simulink model "Actuators"  (Simulink 8.4)
settings: Solver=ode45  StartTime=0.0  StopTime=10.0  RelTol=1e-3
undefined symbols (not defined in the file): Ais_flgAirInjReacPumpOverride, Ais_stAirInjReacPumpMan, Apv_facAirPumpRateMan, Apv_factor, Apv_flgAirPumpRateOverride, Apv_tiPeriod_C, CDRV_E_OK_, Cov_facChOverVlvRateMan, Cov_factor, Cov_flgChOverVlvRateOverride, Cov_tiPeriod_C, Doh_OutputDiagnosisOverride, Fps_flgFuelPumpOverride, Fps_stFuelPumpMan, Icc_degIgnMan, Icc_flgIgnAngleOverride, Icc_flgIgnCutoffMan, Icc_flgIgnCutoffOverride, Icc_nrFollowUpSparks, Icc_tiDwell, Icc_tiDwellFollowUpSparks, Icc_tiOffFollowUpSparks, Ics_flgIntercoolerOverride, Ics_stIntercoolerMan, Ivc_degInjAbort, Ivc_degIntakeClose, Ivc_degOffsetInjEndSimultanInj, Ivc_flgBattDelayOverride, Ivc_flgDiagEntryCondFulfilled, Ivc_flgEndOfStartCond, Ivc_flgInjCutoff, Ivc_flgInjCutoffOverride, Ivc_flgInjTimeOverride, Ivc_flgOverrunCutoff, Ivc_flgPostInjCond, Ivc_tiBattDelayMan, Ivc_tiInjEff, Ivc_tiInjMan, Ivc_tiMinThresDeltaEffInjPeriod, Ivc_weea0, Ivc_weea1, Ivc_weea2, Lo_, Mrs_flgMainRelaisOverride, Mrs_stMainRelaisMan, Normal, OK, OpenCircuit, OverTemp, ShortToBatt, ShortToBattNEG, ShortToGnd, ShortToGndNEG, ShortToGndPOS, Str_flgStarterOverride, Str_stStarterMan, Tvc_facDutycyclePIDLimitMax, Tvc_facDutycyclePIDLimitMin, Tvc_facDutycyclePilotControlNeg, Tvc_facDutycyclePilotControlPos ... (+20)
libraries: simulink x9
(part 2 of 3)

== system Actuators/Actuators_mdl/Apv/G1_PWM_Output_Ctrl ==
  dutycycle : Inport
  period : Inport  Port=2
  factor : Inport  Port=3
  level : Inport  Port=4
  DTC_PwmOut_DutyCycle : DataTypeConversion  OutDataTypeStr=int16  RndMeth=Nearest
  DTC_PwmOut_ErrorInfo : DataTypeConversion  OutDataTypeStr=boolean
  DTC_PwmOut_Level : DataTypeConversion  OutDataTypeStr=int16  RndMeth=Nearest
  DTC_PwmOut_Period : DataTypeConversion  OutDataTypeStr=int16  RndMeth=Nearest
  DTC_PwmOut_Period1 : DataTypeConversion  OutDataTypeStr=uint8  RndMeth=Nearest
  FlexECU_DevLib_FcnAPI_Wrapper_SFcn : S-Function  FunctionName=ehooks_medc17flex_devlib_basic_io_fcncall  Parameters=NoInputPorts, NoOutputPorts, InputPortDataTypes, OutputPortDataTypes, CFunctionArgTypes, CFunctionName, ChannelName  EnableBusSupport=off  mask{NoInputPorts=4, NoOutputPorts=1, InputPortDataTypes=int16,int16, int16, uint8, OutputPortDataTypes=uint8, CFunctionArgTypes=ret,val,val,val,val, CFunctionName=DevLib_Pwm_Out, ChannelName=O_T_RL13}
      mask prompts: NoInputPorts "Number of input ports"; NoOutputPorts "Number of output ports"; InputPortDataTypes "Input port data types"; OutputPortDataTypes "Output port data types"; CFunctionArgTypes "C function argument types"; CFunctionName "C function name"; ChannelName "Channel (pin) name"
      mask Display: disp('EHOOKS FlexECU\nDevLib Wrapper\nS-Function')
  Gain : Gain  Gain=100
  status : Outport
  wires:
  DTC_PwmOut_ErrorInfo/1 -> status/1
  DTC_PwmOut_Level/1 -> FlexECU_DevLib_FcnAPI_Wrapper_SFcn/3
  DTC_PwmOut_Period/1 -> FlexECU_DevLib_FcnAPI_Wrapper_SFcn/2
  DTC_PwmOut_DutyCycle/1 -> FlexECU_DevLib_FcnAPI_Wrapper_SFcn/1
  factor/1 -> DTC_PwmOut_Level/1
  period/1 -> DTC_PwmOut_Period/1
  FlexECU_DevLib_FcnAPI_Wrapper_SFcn/1 -> DTC_PwmOut_ErrorInfo/1
  DTC_PwmOut_Period1/1 -> FlexECU_DevLib_FcnAPI_Wrapper_SFcn/4
  level/1 -> DTC_PwmOut_Period1/1
  dutycycle/1 -> Gain/1
  Gain/1 -> DTC_PwmOut_DutyCycle/1

== system Actuators/Actuators_mdl/Apv/G1_PwmOut_Get_error ==
  DTC_PwmOut_GetError : DataTypeConversion  OutDataTypeStr=single
  FlexECU_DevLib_FcnAPI_Wrapper_SFcn : S-Function  FunctionName=ehooks_medc17flex_devlib_basic_io_fcncall  Parameters=NoInputPorts, NoOutputPorts, InputPortDataTypes, OutputPortDataTypes, CFunctionArgTypes, CFunctionName, ChannelName  EnableBusSupport=off  mask{NoInputPorts=0, NoOutputPorts=1, InputPortDataTypes=, OutputPortDataTypes=uint8, CFunctionArgTypes=ret, CFunctionName=DevLib_PwmOut_GetError, ChannelName=O_T_RL13}
      mask prompts: NoInputPorts "Number of input ports"; NoOutputPorts "Number of output ports"; InputPortDataTypes "Input port data types"; OutputPortDataTypes "Output port data types"; CFunctionArgTypes "C function argument types"; CFunctionName "C function name"; ChannelName "Channel (pin) name"
      mask Display: disp('EHOOKS FlexECU\nDevLib Wrapper\nS-Function')
  status : Outport
  wires:
  FlexECU_DevLib_FcnAPI_Wrapper_SFcn/1 -> DTC_PwmOut_GetError/1
  DTC_PwmOut_GetError/1 -> status/1

== system Actuators/Actuators_mdl/Cov/G1_PWM_Output_Ctrl ==
  dutycycle : Inport
  period : Inport  Port=2
  factor : Inport  Port=3
  level : Inport  Port=4
  DTC_PwmOut_DutyCycle : DataTypeConversion  OutDataTypeStr=int16  RndMeth=Nearest
  DTC_PwmOut_ErrorInfo : DataTypeConversion  OutDataTypeStr=boolean
  DTC_PwmOut_Level : DataTypeConversion  OutDataTypeStr=int16  RndMeth=Nearest
  DTC_PwmOut_Period : DataTypeConversion  OutDataTypeStr=int16  RndMeth=Nearest
  DTC_PwmOut_Period1 : DataTypeConversion  OutDataTypeStr=uint8  RndMeth=Nearest
  FlexECU_DevLib_FcnAPI_Wrapper_SFcn : S-Function  FunctionName=ehooks_medc17flex_devlib_basic_io_fcncall  Parameters=NoInputPorts, NoOutputPorts, InputPortDataTypes, OutputPortDataTypes, CFunctionArgTypes, CFunctionName, ChannelName  EnableBusSupport=off  mask{NoInputPorts=4, NoOutputPorts=1, InputPortDataTypes=int16,int16, int16, uint8, OutputPortDataTypes=uint8, CFunctionArgTypes=ret,val,val,val,val, CFunctionName=DevLib_Pwm_Out, ChannelName=O_T_RL10}
      mask prompts: NoInputPorts "Number of input ports"; NoOutputPorts "Number of output ports"; InputPortDataTypes "Input port data types"; OutputPortDataTypes "Output port data types"; CFunctionArgTypes "C function argument types"; CFunctionName "C function name"; ChannelName "Channel (pin) name"
      mask Display: disp('EHOOKS FlexECU\nDevLib Wrapper\nS-Function')
  Gain : Gain  Gain=100
  status : Outport
  wires:
  Gain/1 -> DTC_PwmOut_DutyCycle/1
  dutycycle/1 -> Gain/1
  level/1 -> DTC_PwmOut_Period1/1
  DTC_PwmOut_Period1/1 -> FlexECU_DevLib_FcnAPI_Wrapper_SFcn/4
  FlexECU_DevLib_FcnAPI_Wrapper_SFcn/1 -> DTC_PwmOut_ErrorInfo/1
  period/1 -> DTC_PwmOut_Period/1
  factor/1 -> DTC_PwmOut_Level/1
  DTC_PwmOut_DutyCycle/1 -> FlexECU_DevLib_FcnAPI_Wrapper_SFcn/1
  DTC_PwmOut_Period/1 -> FlexECU_DevLib_FcnAPI_Wrapper_SFcn/2
  DTC_PwmOut_Level/1 -> FlexECU_DevLib_FcnAPI_Wrapper_SFcn/3
  DTC_PwmOut_ErrorInfo/1 -> status/1

== system Actuators/Actuators_mdl/Cov/G1_PwmOut_Get_error ==
  DTC_PwmOut_GetError : DataTypeConversion  OutDataTypeStr=single
  FlexECU_DevLib_FcnAPI_Wrapper_SFcn : S-Function  FunctionName=ehooks_medc17flex_devlib_basic_io_fcncall  Parameters=NoInputPorts, NoOutputPorts, InputPortDataTypes, OutputPortDataTypes, CFunctionArgTypes, CFunctionName, ChannelName  EnableBusSupport=off  mask{NoInputPorts=0, NoOutputPorts=1, InputPortDataTypes=, OutputPortDataTypes=uint8, CFunctionArgTypes=ret, CFunctionName=DevLib_PwmOut_GetError, ChannelName=O_T_RL10}
      mask prompts: NoInputPorts "Number of input ports"; NoOutputPorts "Number of output ports"; InputPortDataTypes "Input port data types"; OutputPortDataTypes "Output port data types"; CFunctionArgTypes "C function argument types"; CFunctionName "C function name"; ChannelName "Channel (pin) name"
      mask Display: disp('EHOOKS FlexECU\nDevLib Wrapper\nS-Function')
  status : Outport
  wires:
  DTC_PwmOut_GetError/1 -> status/1
  FlexECU_DevLib_FcnAPI_Wrapper_SFcn/1 -> DTC_PwmOut_GetError/1

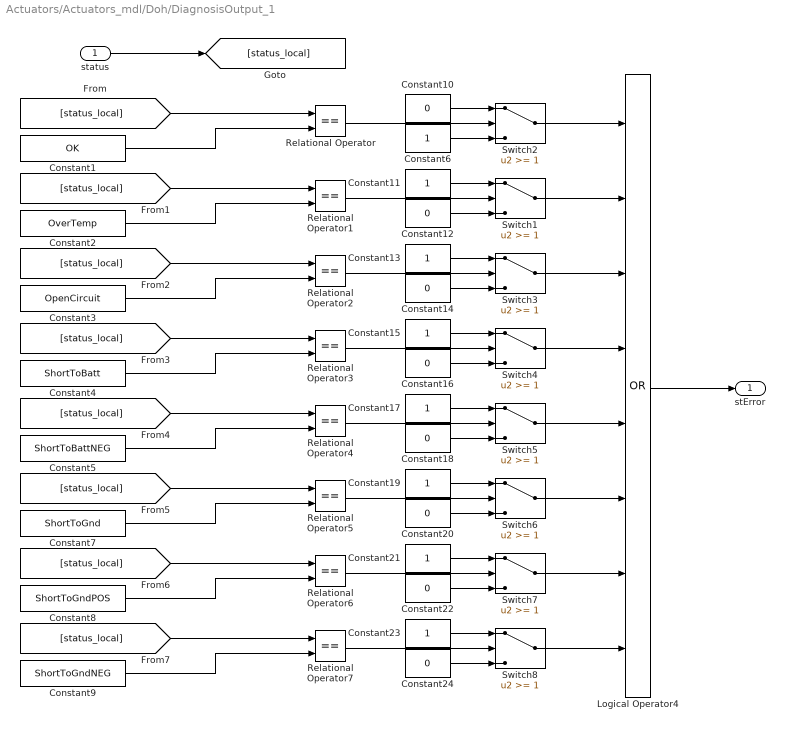
== system Actuators/Actuators_mdl/Doh/DiagnosisOutput_1 ==
  status : Inport
  Constant1 : Constant  Value=OK
  Constant{10,12,14,16,18,20,22,24} (8 alike) : Constant  Value=0  OutDataTypeStr=boolean
  Constant{6,11,13,15,17,19,21,23} (8 alike) : Constant  OutDataTypeStr=boolean
  Constant2 : Constant  Value=OverTemp
  Constant3 : Constant  Value=OpenCircuit
  Constant4 : Constant  Value=ShortToBatt
  Constant5 : Constant  Value=ShortToBattNEG
  Constant7 : Constant  Value=ShortToGnd
  Constant8 : Constant  Value=ShortToGndPOS
  Constant9 : Constant  Value=ShortToGndNEG
  Logical Operator4 : Logic  Operator=OR  Inputs=8  AllPortsSameDT=off  OutDataTypeStr=boolean
  Relational Operator{,1..7} (8 alike) : RelationalOperator  Operator===  OutDataTypeStr=boolean
  Switch{1..8} (8 alike) : Switch  Threshold=1
  stError : Outport
  wires:
  Constant1/1 -> Relational Operator/2
  status/1 -> [status_local]
  [status_local] -> Relational Operator/1
  Constant2/1 -> Relational Operator1/2
  [status_local] -> Relational Operator1/1
  Constant3/1 -> Relational Operator2/2
  [status_local] -> Relational Operator2/1
  Constant4/1 -> Relational Operator3/2
  [status_local] -> Relational Operator3/1
  Constant5/1 -> Relational Operator4/2
  [status_local] -> Relational Operator4/1
  Constant7/1 -> Relational Operator5/2
  [status_local] -> Relational Operator5/1
  Constant8/1 -> Relational Operator6/2
  [status_local] -> Relational Operator6/1
  Constant9/1 -> Relational Operator7/2
  [status_local] -> Relational Operator7/1
  Relational Operator/1 -> Switch2/2
  Constant6/1 -> Switch2/3
  Logical Operator4/1 -> stError/1
  Constant10/1 -> Switch2/1
  Constant12/1 -> Switch1/3
  Constant11/1 -> Switch1/1
  Relational Operator1/1 -> Switch1/2
  Constant14/1 -> Switch3/3
  Constant13/1 -> Switch3/1
  Relational Operator2/1 -> Switch3/2
  Constant16/1 -> Switch4/3
  Constant15/1 -> Switch4/1
  Relational Operator3/1 -> Switch4/2
  Constant18/1 -> Switch5/3
  Constant17/1 -> Switch5/1
  Relational Operator4/1 -> Switch5/2
  Constant20/1 -> Switch6/3
  Constant19/1 -> Switch6/1
  Relational Operator5/1 -> Switch6/2
  Constant22/1 -> Switch7/3
  Constant21/1 -> Switch7/1
  Relational Operator6/1 -> Switch7/2
  Constant24/1 -> Switch8/3
  Constant23/1 -> Switch8/1
  Relational Operator7/1 -> Switch8/2
  Switch2/1 -> Logical Operator4/1
  Switch1/1 -> Logical Operator4/2
  Switch3/1 -> Logical Operator4/3
  Switch4/1 -> Logical Operator4/4
  Switch5/1 -> Logical Operator4/5
  Switch6/1 -> Logical Operator4/6
  Switch7/1 -> Logical Operator4/7
  Switch8/1 -> Logical Operator4/8

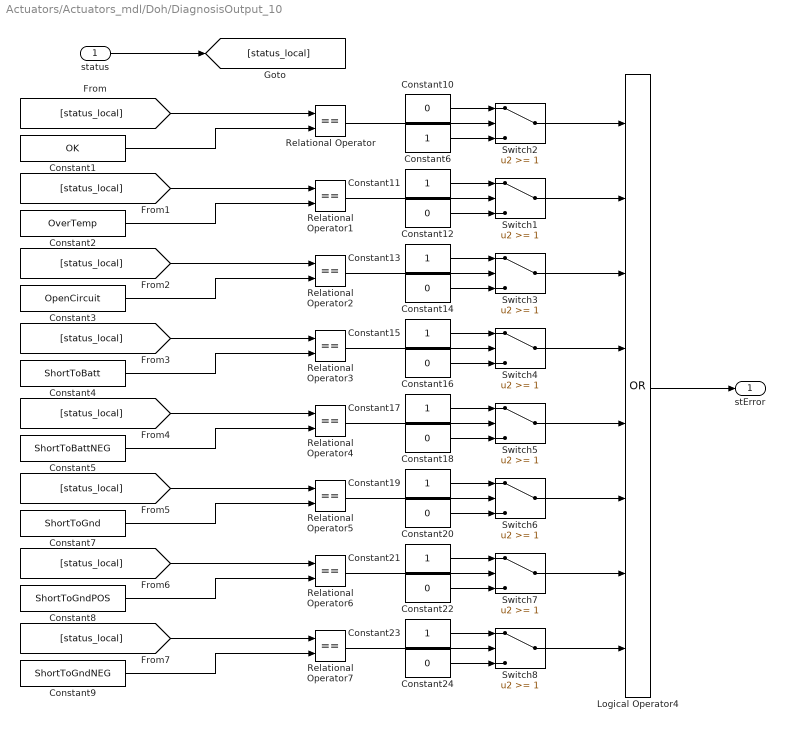
== system Actuators/Actuators_mdl/Doh/DiagnosisOutput_10 ==
  status : Inport
  Constant1 : Constant  Value=OK
  Constant{10,12,14,16,18,20,22,24} (8 alike) : Constant  Value=0  OutDataTypeStr=boolean
  Constant{6,11,13,15,17,19,21,23} (8 alike) : Constant  OutDataTypeStr=boolean
  Constant2 : Constant  Value=OverTemp
  Constant3 : Constant  Value=OpenCircuit
  Constant4 : Constant  Value=ShortToBatt
  Constant5 : Constant  Value=ShortToBattNEG
  Constant7 : Constant  Value=ShortToGnd
  Constant8 : Constant  Value=ShortToGndPOS
  Constant9 : Constant  Value=ShortToGndNEG
  Logical Operator4 : Logic  Operator=OR  Inputs=8  AllPortsSameDT=off  OutDataTypeStr=boolean
  Relational Operator{,1..7} (8 alike) : RelationalOperator  Operator===  OutDataTypeStr=boolean
  Switch{1..8} (8 alike) : Switch  Threshold=1
  stError : Outport
  wires:
  Switch8/1 -> Logical Operator4/8
  Switch7/1 -> Logical Operator4/7
  Switch6/1 -> Logical Operator4/6
  Switch5/1 -> Logical Operator4/5
  Switch4/1 -> Logical Operator4/4
  Switch3/1 -> Logical Operator4/3
  Switch1/1 -> Logical Operator4/2
  Switch2/1 -> Logical Operator4/1
  Relational Operator7/1 -> Switch8/2
  Constant23/1 -> Switch8/1
  Constant24/1 -> Switch8/3
  Relational Operator6/1 -> Switch7/2
  Constant21/1 -> Switch7/1
  Constant22/1 -> Switch7/3
  Relational Operator5/1 -> Switch6/2
  Constant19/1 -> Switch6/1
  Constant20/1 -> Switch6/3
  Relational Operator4/1 -> Switch5/2
  Constant17/1 -> Switch5/1
  Constant18/1 -> Switch5/3
  Relational Operator3/1 -> Switch4/2
  Constant15/1 -> Switch4/1
  Constant16/1 -> Switch4/3
  Relational Operator2/1 -> Switch3/2
  Constant13/1 -> Switch3/1
  Constant14/1 -> Switch3/3
  Relational Operator1/1 -> Switch1/2
  Constant11/1 -> Switch1/1
  Constant12/1 -> Switch1/3
  Constant10/1 -> Switch2/1
  Logical Operator4/1 -> stError/1
  Constant6/1 -> Switch2/3
  Relational Operator/1 -> Switch2/2
  [status_local] -> Relational Operator7/1
  Constant9/1 -> Relational Operator7/2
  [status_local] -> Relational Operator6/1
  Constant8/1 -> Relational Operator6/2
  [status_local] -> Relational Operator5/1
  Constant7/1 -> Relational Operator5/2
  [status_local] -> Relational Operator4/1
  Constant5/1 -> Relational Operator4/2
  [status_local] -> Relational Operator3/1
  Constant4/1 -> Relational Operator3/2
  [status_local] -> Relational Operator2/1
  Constant3/1 -> Relational Operator2/2
  [status_local] -> Relational Operator1/1
  Constant2/1 -> Relational Operator1/2
  [status_local] -> Relational Operator/1
  status/1 -> [status_local]
  Constant1/1 -> Relational Operator/2

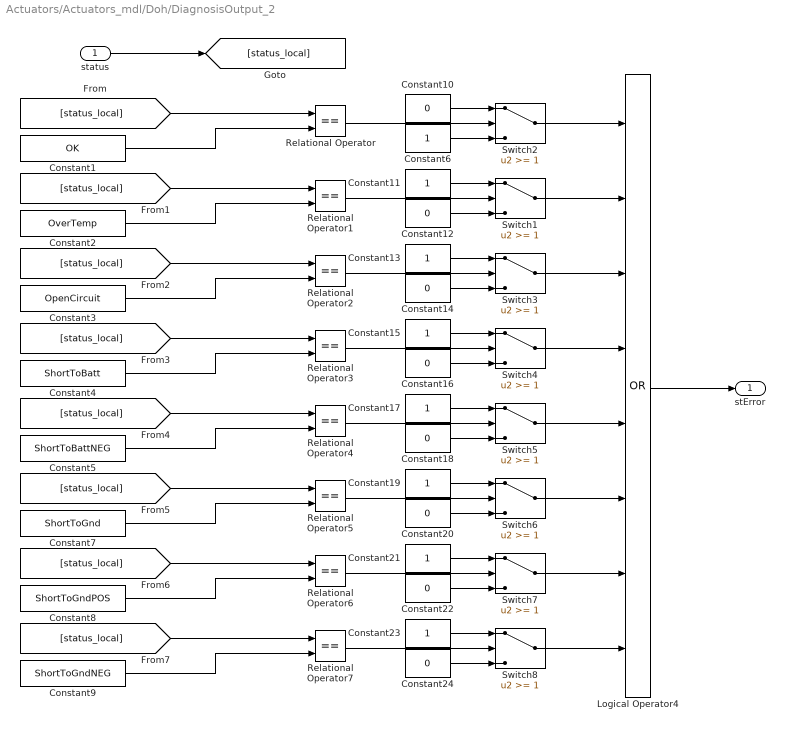
== system Actuators/Actuators_mdl/Doh/DiagnosisOutput_2 ==
  status : Inport
  Constant1 : Constant  Value=OK
  Constant{10,12,14,16,18,20,22,24} (8 alike) : Constant  Value=0  OutDataTypeStr=boolean
  Constant{6,11,13,15,17,19,21,23} (8 alike) : Constant  OutDataTypeStr=boolean
  Constant2 : Constant  Value=OverTemp
  Constant3 : Constant  Value=OpenCircuit
  Constant4 : Constant  Value=ShortToBatt
  Constant5 : Constant  Value=ShortToBattNEG
  Constant7 : Constant  Value=ShortToGnd
  Constant8 : Constant  Value=ShortToGndPOS
  Constant9 : Constant  Value=ShortToGndNEG
  Logical Operator4 : Logic  Operator=OR  Inputs=8  AllPortsSameDT=off  OutDataTypeStr=boolean
  Relational Operator{,1..7} (8 alike) : RelationalOperator  Operator===  OutDataTypeStr=boolean
  Switch{1..8} (8 alike) : Switch  Threshold=1
  stError : Outport
  wires:
  Switch8/1 -> Logical Operator4/8
  Switch7/1 -> Logical Operator4/7
  Switch6/1 -> Logical Operator4/6
  Switch5/1 -> Logical Operator4/5
  Switch4/1 -> Logical Operator4/4
  Switch3/1 -> Logical Operator4/3
  Switch1/1 -> Logical Operator4/2
  Switch2/1 -> Logical Operator4/1
  Relational Operator7/1 -> Switch8/2
  Constant23/1 -> Switch8/1
  Constant24/1 -> Switch8/3
  Relational Operator6/1 -> Switch7/2
  Constant21/1 -> Switch7/1
  Constant22/1 -> Switch7/3
  Relational Operator5/1 -> Switch6/2
  Constant19/1 -> Switch6/1
  Constant20/1 -> Switch6/3
  Relational Operator4/1 -> Switch5/2
  Constant17/1 -> Switch5/1
  Constant18/1 -> Switch5/3
  Relational Operator3/1 -> Switch4/2
  Constant15/1 -> Switch4/1
  Constant16/1 -> Switch4/3
  Relational Operator2/1 -> Switch3/2
  Constant13/1 -> Switch3/1
  Constant14/1 -> Switch3/3
  Relational Operator1/1 -> Switch1/2
  Constant11/1 -> Switch1/1
  Constant12/1 -> Switch1/3
  Constant10/1 -> Switch2/1
  Logical Operator4/1 -> stError/1
  Constant6/1 -> Switch2/3
  Relational Operator/1 -> Switch2/2
  [status_local] -> Relational Operator7/1
  Constant9/1 -> Relational Operator7/2
  [status_local] -> Relational Operator6/1
  Constant8/1 -> Relational Operator6/2
  [status_local] -> Relational Operator5/1
  Constant7/1 -> Relational Operator5/2
  [status_local] -> Relational Operator4/1
  Constant5/1 -> Relational Operator4/2
  [status_local] -> Relational Operator3/1
  Constant4/1 -> Relational Operator3/2
  [status_local] -> Relational Operator2/1
  Constant3/1 -> Relational Operator2/2
  [status_local] -> Relational Operator1/1
  Constant2/1 -> Relational Operator1/2
  [status_local] -> Relational Operator/1
  status/1 -> [status_local]
  Constant1/1 -> Relational Operator/2

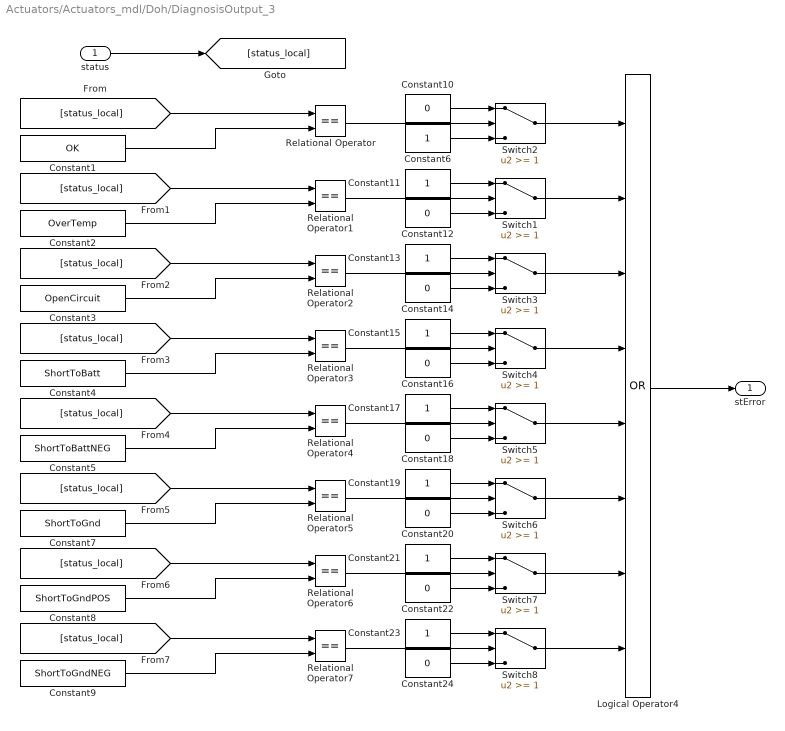
== system Actuators/Actuators_mdl/Doh/DiagnosisOutput_3 ==
  status : Inport
  Constant1 : Constant  Value=OK
  Constant{10,12,14,16,18,20,22,24} (8 alike) : Constant  Value=0  OutDataTypeStr=boolean
  Constant{6,11,13,15,17,19,21,23} (8 alike) : Constant  OutDataTypeStr=boolean
  Constant2 : Constant  Value=OverTemp
  Constant3 : Constant  Value=OpenCircuit
  Constant4 : Constant  Value=ShortToBatt
  Constant5 : Constant  Value=ShortToBattNEG
  Constant7 : Constant  Value=ShortToGnd
  Constant8 : Constant  Value=ShortToGndPOS
  Constant9 : Constant  Value=ShortToGndNEG
  Logical Operator4 : Logic  Operator=OR  Inputs=8  AllPortsSameDT=off  OutDataTypeStr=boolean
  Relational Operator{,1..7} (8 alike) : RelationalOperator  Operator===  OutDataTypeStr=boolean
  Switch{1..8} (8 alike) : Switch  Threshold=1
  stError : Outport
  wires:
  Constant1/1 -> Relational Operator/2
  status/1 -> [status_local]
  [status_local] -> Relational Operator/1
  Constant2/1 -> Relational Operator1/2
  [status_local] -> Relational Operator1/1
  Constant3/1 -> Relational Operator2/2
  [status_local] -> Relational Operator2/1
  Constant4/1 -> Relational Operator3/2
  [status_local] -> Relational Operator3/1
  Constant5/1 -> Relational Operator4/2
  [status_local] -> Relational Operator4/1
  Constant7/1 -> Relational Operator5/2
  [status_local] -> Relational Operator5/1
  Constant8/1 -> Relational Operator6/2
  [status_local] -> Relational Operator6/1
  Constant9/1 -> Relational Operator7/2
  [status_local] -> Relational Operator7/1
  Relational Operator/1 -> Switch2/2
  Constant6/1 -> Switch2/3
  Logical Operator4/1 -> stError/1
  Constant10/1 -> Switch2/1
  Constant12/1 -> Switch1/3
  Constant11/1 -> Switch1/1
  Relational Operator1/1 -> Switch1/2
  Constant14/1 -> Switch3/3
  Constant13/1 -> Switch3/1
  Relational Operator2/1 -> Switch3/2
  Constant16/1 -> Switch4/3
  Constant15/1 -> Switch4/1
  Relational Operator3/1 -> Switch4/2
  Constant18/1 -> Switch5/3
  Constant17/1 -> Switch5/1
  Relational Operator4/1 -> Switch5/2
  Constant20/1 -> Switch6/3
  Constant19/1 -> Switch6/1
  Relational Operator5/1 -> Switch6/2
  Constant22/1 -> Switch7/3
  Constant21/1 -> Switch7/1
  Relational Operator6/1 -> Switch7/2
  Constant24/1 -> Switch8/3
  Constant23/1 -> Switch8/1
  Relational Operator7/1 -> Switch8/2
  Switch2/1 -> Logical Operator4/1
  Switch1/1 -> Logical Operator4/2
  Switch3/1 -> Logical Operator4/3
  Switch4/1 -> Logical Operator4/4
  Switch5/1 -> Logical Operator4/5
  Switch6/1 -> Logical Operator4/6
  Switch7/1 -> Logical Operator4/7
  Switch8/1 -> Logical Operator4/8

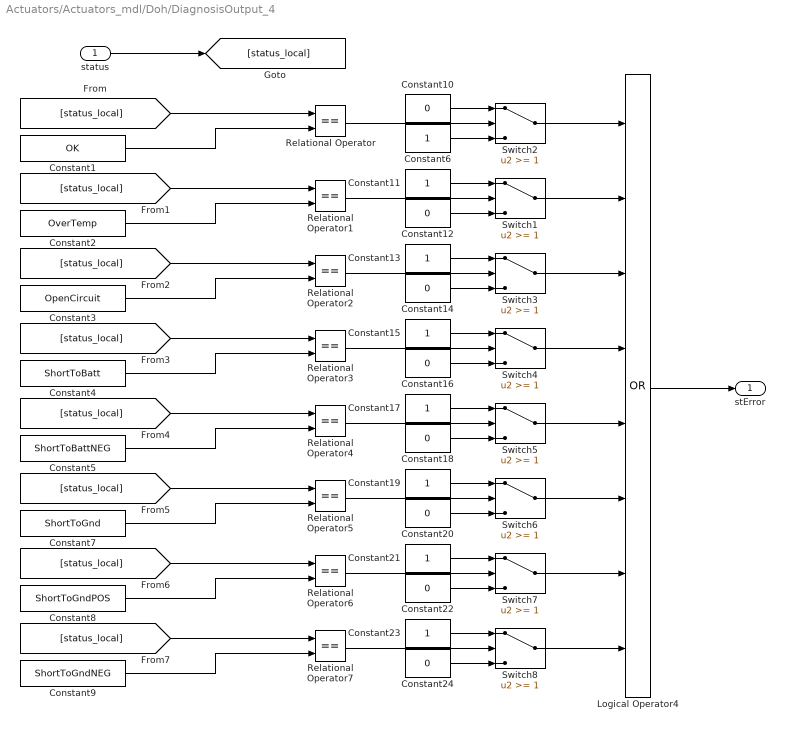
== system Actuators/Actuators_mdl/Doh/DiagnosisOutput_4 ==
  status : Inport
  Constant1 : Constant  Value=OK
  Constant{10,12,14,16,18,20,22,24} (8 alike) : Constant  Value=0  OutDataTypeStr=boolean
  Constant{6,11,13,15,17,19,21,23} (8 alike) : Constant  OutDataTypeStr=boolean
  Constant2 : Constant  Value=OverTemp
  Constant3 : Constant  Value=OpenCircuit
  Constant4 : Constant  Value=ShortToBatt
  Constant5 : Constant  Value=ShortToBattNEG
  Constant7 : Constant  Value=ShortToGnd
  Constant8 : Constant  Value=ShortToGndPOS
  Constant9 : Constant  Value=ShortToGndNEG
  Logical Operator4 : Logic  Operator=OR  Inputs=8  AllPortsSameDT=off  OutDataTypeStr=boolean
  Relational Operator{,1..7} (8 alike) : RelationalOperator  Operator===  OutDataTypeStr=boolean
  Switch{1..8} (8 alike) : Switch  Threshold=1
  stError : Outport
  wires:
  Switch8/1 -> Logical Operator4/8
  Switch7/1 -> Logical Operator4/7
  Switch6/1 -> Logical Operator4/6
  Switch5/1 -> Logical Operator4/5
  Switch4/1 -> Logical Operator4/4
  Switch3/1 -> Logical Operator4/3
  Switch1/1 -> Logical Operator4/2
  Switch2/1 -> Logical Operator4/1
  Relational Operator7/1 -> Switch8/2
  Constant23/1 -> Switch8/1
  Constant24/1 -> Switch8/3
  Relational Operator6/1 -> Switch7/2
  Constant21/1 -> Switch7/1
  Constant22/1 -> Switch7/3
  Relational Operator5/1 -> Switch6/2
  Constant19/1 -> Switch6/1
  Constant20/1 -> Switch6/3
  Relational Operator4/1 -> Switch5/2
  Constant17/1 -> Switch5/1
  Constant18/1 -> Switch5/3
  Relational Operator3/1 -> Switch4/2
  Constant15/1 -> Switch4/1
  Constant16/1 -> Switch4/3
  Relational Operator2/1 -> Switch3/2
  Constant13/1 -> Switch3/1
  Constant14/1 -> Switch3/3
  Relational Operator1/1 -> Switch1/2
  Constant11/1 -> Switch1/1
  Constant12/1 -> Switch1/3
  Constant10/1 -> Switch2/1
  Logical Operator4/1 -> stError/1
  Constant6/1 -> Switch2/3
  Relational Operator/1 -> Switch2/2
  [status_local] -> Relational Operator7/1
  Constant9/1 -> Relational Operator7/2
  [status_local] -> Relational Operator6/1
  Constant8/1 -> Relational Operator6/2
  [status_local] -> Relational Operator5/1
  Constant7/1 -> Relational Operator5/2
  [status_local] -> Relational Operator4/1
  Constant5/1 -> Relational Operator4/2
  [status_local] -> Relational Operator3/1
  Constant4/1 -> Relational Operator3/2
  [status_local] -> Relational Operator2/1
  Constant3/1 -> Relational Operator2/2
  [status_local] -> Relational Operator1/1
  Constant2/1 -> Relational Operator1/2
  [status_local] -> Relational Operator/1
  status/1 -> [status_local]
  Constant1/1 -> Relational Operator/2

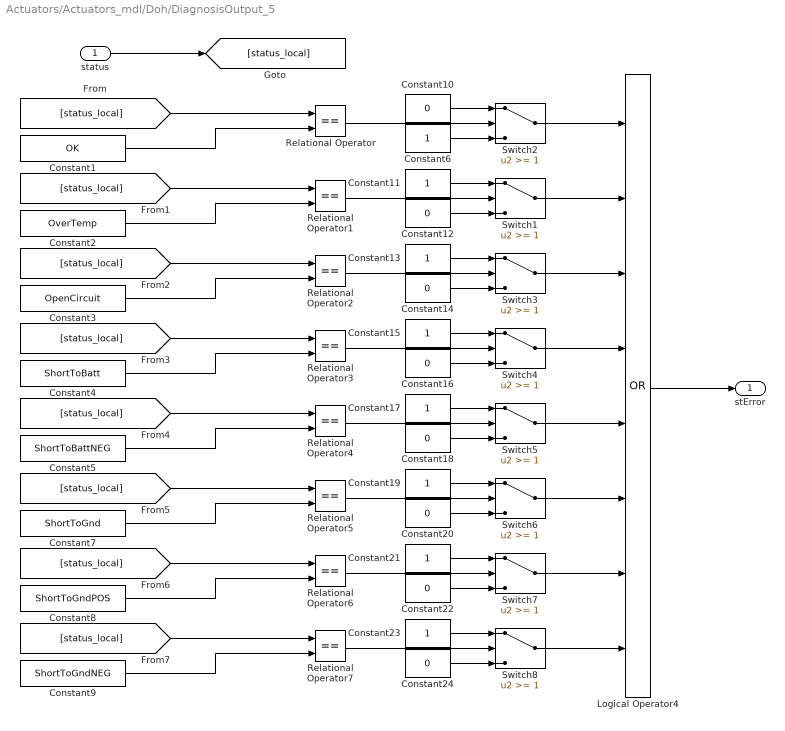
== system Actuators/Actuators_mdl/Doh/DiagnosisOutput_5 ==
  status : Inport
  Constant1 : Constant  Value=OK
  Constant{10,12,14,16,18,20,22,24} (8 alike) : Constant  Value=0  OutDataTypeStr=boolean
  Constant{6,11,13,15,17,19,21,23} (8 alike) : Constant  OutDataTypeStr=boolean
  Constant2 : Constant  Value=OverTemp
  Constant3 : Constant  Value=OpenCircuit
  Constant4 : Constant  Value=ShortToBatt
  Constant5 : Constant  Value=ShortToBattNEG
  Constant7 : Constant  Value=ShortToGnd
  Constant8 : Constant  Value=ShortToGndPOS
  Constant9 : Constant  Value=ShortToGndNEG
  Logical Operator4 : Logic  Operator=OR  Inputs=8  AllPortsSameDT=off  OutDataTypeStr=boolean
  Relational Operator{,1..7} (8 alike) : RelationalOperator  Operator===  OutDataTypeStr=boolean
  Switch{1..8} (8 alike) : Switch  Threshold=1
  stError : Outport
  wires:
  Constant1/1 -> Relational Operator/2
  status/1 -> [status_local]
  [status_local] -> Relational Operator/1
  Constant2/1 -> Relational Operator1/2
  [status_local] -> Relational Operator1/1
  Constant3/1 -> Relational Operator2/2
  [status_local] -> Relational Operator2/1
  Constant4/1 -> Relational Operator3/2
  [status_local] -> Relational Operator3/1
  Constant5/1 -> Relational Operator4/2
  [status_local] -> Relational Operator4/1
  Constant7/1 -> Relational Operator5/2
  [status_local] -> Relational Operator5/1
  Constant8/1 -> Relational Operator6/2
  [status_local] -> Relational Operator6/1
  Constant9/1 -> Relational Operator7/2
  [status_local] -> Relational Operator7/1
  Relational Operator/1 -> Switch2/2
  Constant6/1 -> Switch2/3
  Logical Operator4/1 -> stError/1
  Constant10/1 -> Switch2/1
  Constant12/1 -> Switch1/3
  Constant11/1 -> Switch1/1
  Relational Operator1/1 -> Switch1/2
  Constant14/1 -> Switch3/3
  Constant13/1 -> Switch3/1
  Relational Operator2/1 -> Switch3/2
  Constant16/1 -> Switch4/3
  Constant15/1 -> Switch4/1
  Relational Operator3/1 -> Switch4/2
  Constant18/1 -> Switch5/3
  Constant17/1 -> Switch5/1
  Relational Operator4/1 -> Switch5/2
  Constant20/1 -> Switch6/3
  Constant19/1 -> Switch6/1
  Relational Operator5/1 -> Switch6/2
  Constant22/1 -> Switch7/3
  Constant21/1 -> Switch7/1
  Relational Operator6/1 -> Switch7/2
  Constant24/1 -> Switch8/3
  Constant23/1 -> Switch8/1
  Relational Operator7/1 -> Switch8/2
  Switch2/1 -> Logical Operator4/1
  Switch1/1 -> Logical Operator4/2
  Switch3/1 -> Logical Operator4/3
  Switch4/1 -> Logical Operator4/4
  Switch5/1 -> Logical Operator4/5
  Switch6/1 -> Logical Operator4/6
  Switch7/1 -> Logical Operator4/7
  Switch8/1 -> Logical Operator4/8

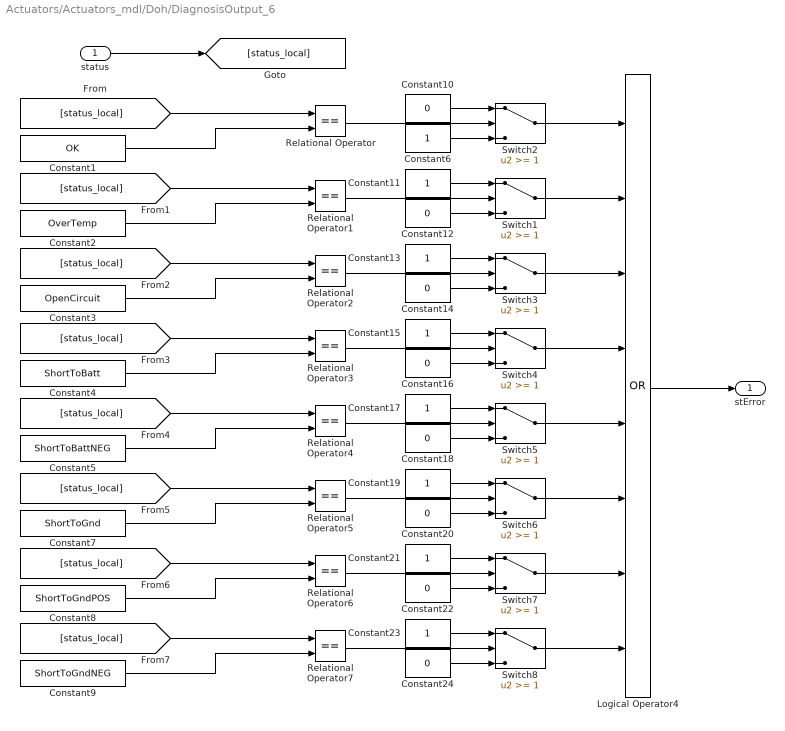
== system Actuators/Actuators_mdl/Doh/DiagnosisOutput_6 ==
  status : Inport
  Constant1 : Constant  Value=OK
  Constant{10,12,14,16,18,20,22,24} (8 alike) : Constant  Value=0  OutDataTypeStr=boolean
  Constant{6,11,13,15,17,19,21,23} (8 alike) : Constant  OutDataTypeStr=boolean
  Constant2 : Constant  Value=OverTemp
  Constant3 : Constant  Value=OpenCircuit
  Constant4 : Constant  Value=ShortToBatt
  Constant5 : Constant  Value=ShortToBattNEG
  Constant7 : Constant  Value=ShortToGnd
  Constant8 : Constant  Value=ShortToGndPOS
  Constant9 : Constant  Value=ShortToGndNEG
  Logical Operator4 : Logic  Operator=OR  Inputs=8  AllPortsSameDT=off  OutDataTypeStr=boolean
  Relational Operator{,1..7} (8 alike) : RelationalOperator  Operator===  OutDataTypeStr=boolean
  Switch{1..8} (8 alike) : Switch  Threshold=1
  stError : Outport
  wires:
  Switch8/1 -> Logical Operator4/8
  Switch7/1 -> Logical Operator4/7
  Switch6/1 -> Logical Operator4/6
  Switch5/1 -> Logical Operator4/5
  Switch4/1 -> Logical Operator4/4
  Switch3/1 -> Logical Operator4/3
  Switch1/1 -> Logical Operator4/2
  Switch2/1 -> Logical Operator4/1
  Relational Operator7/1 -> Switch8/2
  Constant23/1 -> Switch8/1
  Constant24/1 -> Switch8/3
  Relational Operator6/1 -> Switch7/2
  Constant21/1 -> Switch7/1
  Constant22/1 -> Switch7/3
  Relational Operator5/1 -> Switch6/2
  Constant19/1 -> Switch6/1
  Constant20/1 -> Switch6/3
  Relational Operator4/1 -> Switch5/2
  Constant17/1 -> Switch5/1
  Constant18/1 -> Switch5/3
  Relational Operator3/1 -> Switch4/2
  Constant15/1 -> Switch4/1
  Constant16/1 -> Switch4/3
  Relational Operator2/1 -> Switch3/2
  Constant13/1 -> Switch3/1
  Constant14/1 -> Switch3/3
  Relational Operator1/1 -> Switch1/2
  Constant11/1 -> Switch1/1
  Constant12/1 -> Switch1/3
  Constant10/1 -> Switch2/1
  Logical Operator4/1 -> stError/1
  Constant6/1 -> Switch2/3
  Relational Operator/1 -> Switch2/2
  [status_local] -> Relational Operator7/1
  Constant9/1 -> Relational Operator7/2
  [status_local] -> Relational Operator6/1
  Constant8/1 -> Relational Operator6/2
  [status_local] -> Relational Operator5/1
  Constant7/1 -> Relational Operator5/2
  [status_local] -> Relational Operator4/1
  Constant5/1 -> Relational Operator4/2
  [status_local] -> Relational Operator3/1
  Constant4/1 -> Relational Operator3/2
  [status_local] -> Relational Operator2/1
  Constant3/1 -> Relational Operator2/2
  [status_local] -> Relational Operator1/1
  Constant2/1 -> Relational Operator1/2
  [status_local] -> Relational Operator/1
  status/1 -> [status_local]
  Constant1/1 -> Relational Operator/2

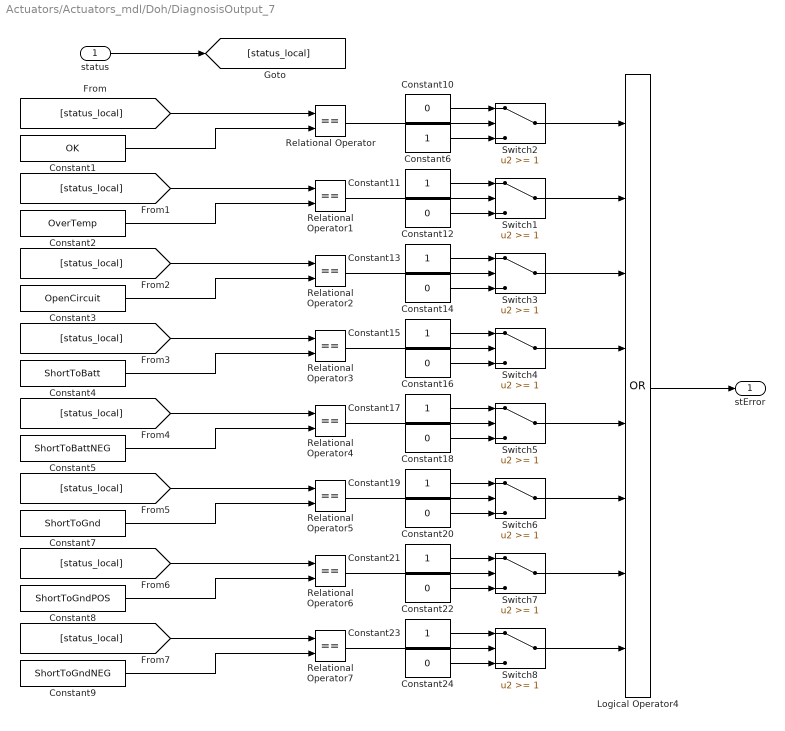
== system Actuators/Actuators_mdl/Doh/DiagnosisOutput_7 ==
  status : Inport
  Constant1 : Constant  Value=OK
  Constant{10,12,14,16,18,20,22,24} (8 alike) : Constant  Value=0  OutDataTypeStr=boolean
  Constant{6,11,13,15,17,19,21,23} (8 alike) : Constant  OutDataTypeStr=boolean
  Constant2 : Constant  Value=OverTemp
  Constant3 : Constant  Value=OpenCircuit
  Constant4 : Constant  Value=ShortToBatt
  Constant5 : Constant  Value=ShortToBattNEG
  Constant7 : Constant  Value=ShortToGnd
  Constant8 : Constant  Value=ShortToGndPOS
  Constant9 : Constant  Value=ShortToGndNEG
  Logical Operator4 : Logic  Operator=OR  Inputs=8  AllPortsSameDT=off  OutDataTypeStr=boolean
  Relational Operator{,1..7} (8 alike) : RelationalOperator  Operator===  OutDataTypeStr=boolean
  Switch{1..8} (8 alike) : Switch  Threshold=1
  stError : Outport
  wires:
  Constant1/1 -> Relational Operator/2
  status/1 -> [status_local]
  [status_local] -> Relational Operator/1
  Constant2/1 -> Relational Operator1/2
  [status_local] -> Relational Operator1/1
  Constant3/1 -> Relational Operator2/2
  [status_local] -> Relational Operator2/1
  Constant4/1 -> Relational Operator3/2
  [status_local] -> Relational Operator3/1
  Constant5/1 -> Relational Operator4/2
  [status_local] -> Relational Operator4/1
  Constant7/1 -> Relational Operator5/2
  [status_local] -> Relational Operator5/1
  Constant8/1 -> Relational Operator6/2
  [status_local] -> Relational Operator6/1
  Constant9/1 -> Relational Operator7/2
  [status_local] -> Relational Operator7/1
  Relational Operator/1 -> Switch2/2
  Constant6/1 -> Switch2/3
  Logical Operator4/1 -> stError/1
  Constant10/1 -> Switch2/1
  Constant12/1 -> Switch1/3
  Constant11/1 -> Switch1/1
  Relational Operator1/1 -> Switch1/2
  Constant14/1 -> Switch3/3
  Constant13/1 -> Switch3/1
  Relational Operator2/1 -> Switch3/2
  Constant16/1 -> Switch4/3
  Constant15/1 -> Switch4/1
  Relational Operator3/1 -> Switch4/2
  Constant18/1 -> Switch5/3
  Constant17/1 -> Switch5/1
  Relational Operator4/1 -> Switch5/2
  Constant20/1 -> Switch6/3
  Constant19/1 -> Switch6/1
  Relational Operator5/1 -> Switch6/2
  Constant22/1 -> Switch7/3
  Constant21/1 -> Switch7/1
  Relational Operator6/1 -> Switch7/2
  Constant24/1 -> Switch8/3
  Constant23/1 -> Switch8/1
  Relational Operator7/1 -> Switch8/2
  Switch2/1 -> Logical Operator4/1
  Switch1/1 -> Logical Operator4/2
  Switch3/1 -> Logical Operator4/3
  Switch4/1 -> Logical Operator4/4
  Switch5/1 -> Logical Operator4/5
  Switch6/1 -> Logical Operator4/6
  Switch7/1 -> Logical Operator4/7
  Switch8/1 -> Logical Operator4/8

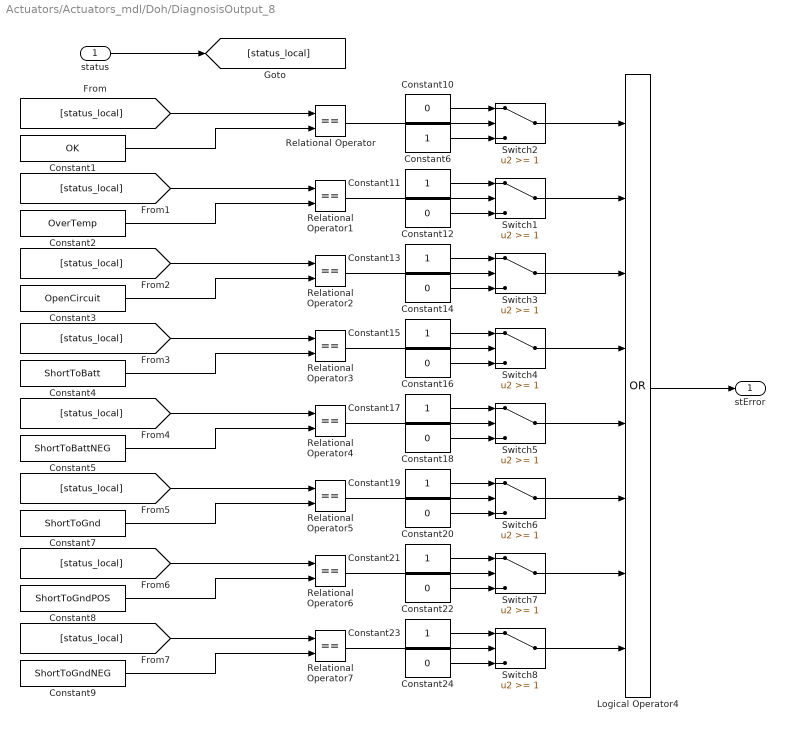
== system Actuators/Actuators_mdl/Doh/DiagnosisOutput_8 ==
  status : Inport
  Constant1 : Constant  Value=OK
  Constant{10,12,14,16,18,20,22,24} (8 alike) : Constant  Value=0  OutDataTypeStr=boolean
  Constant{6,11,13,15,17,19,21,23} (8 alike) : Constant  OutDataTypeStr=boolean
  Constant2 : Constant  Value=OverTemp
  Constant3 : Constant  Value=OpenCircuit
  Constant4 : Constant  Value=ShortToBatt
  Constant5 : Constant  Value=ShortToBattNEG
  Constant7 : Constant  Value=ShortToGnd
  Constant8 : Constant  Value=ShortToGndPOS
  Constant9 : Constant  Value=ShortToGndNEG
  Logical Operator4 : Logic  Operator=OR  Inputs=8  AllPortsSameDT=off  OutDataTypeStr=boolean
  Relational Operator{,1..7} (8 alike) : RelationalOperator  Operator===  OutDataTypeStr=boolean
  Switch{1..8} (8 alike) : Switch  Threshold=1
  stError : Outport
  wires:
  Switch8/1 -> Logical Operator4/8
  Switch7/1 -> Logical Operator4/7
  Switch6/1 -> Logical Operator4/6
  Switch5/1 -> Logical Operator4/5
  Switch4/1 -> Logical Operator4/4
  Switch3/1 -> Logical Operator4/3
  Switch1/1 -> Logical Operator4/2
  Switch2/1 -> Logical Operator4/1
  Relational Operator7/1 -> Switch8/2
  Constant23/1 -> Switch8/1
  Constant24/1 -> Switch8/3
  Relational Operator6/1 -> Switch7/2
  Constant21/1 -> Switch7/1
  Constant22/1 -> Switch7/3
  Relational Operator5/1 -> Switch6/2
  Constant19/1 -> Switch6/1
  Constant20/1 -> Switch6/3
  Relational Operator4/1 -> Switch5/2
  Constant17/1 -> Switch5/1
  Constant18/1 -> Switch5/3
  Relational Operator3/1 -> Switch4/2
  Constant15/1 -> Switch4/1
  Constant16/1 -> Switch4/3
  Relational Operator2/1 -> Switch3/2
  Constant13/1 -> Switch3/1
  Constant14/1 -> Switch3/3
  Relational Operator1/1 -> Switch1/2
  Constant11/1 -> Switch1/1
  Constant12/1 -> Switch1/3
  Constant10/1 -> Switch2/1
  Logical Operator4/1 -> stError/1
  Constant6/1 -> Switch2/3
  Relational Operator/1 -> Switch2/2
  [status_local] -> Relational Operator7/1
  Constant9/1 -> Relational Operator7/2
  [status_local] -> Relational Operator6/1
  Constant8/1 -> Relational Operator6/2
  [status_local] -> Relational Operator5/1
  Constant7/1 -> Relational Operator5/2
  [status_local] -> Relational Operator4/1
  Constant5/1 -> Relational Operator4/2
  [status_local] -> Relational Operator3/1
  Constant4/1 -> Relational Operator3/2
  [status_local] -> Relational Operator2/1
  Constant3/1 -> Relational Operator2/2
  [status_local] -> Relational Operator1/1
  Constant2/1 -> Relational Operator1/2
  [status_local] -> Relational Operator/1
  status/1 -> [status_local]
  Constant1/1 -> Relational Operator/2

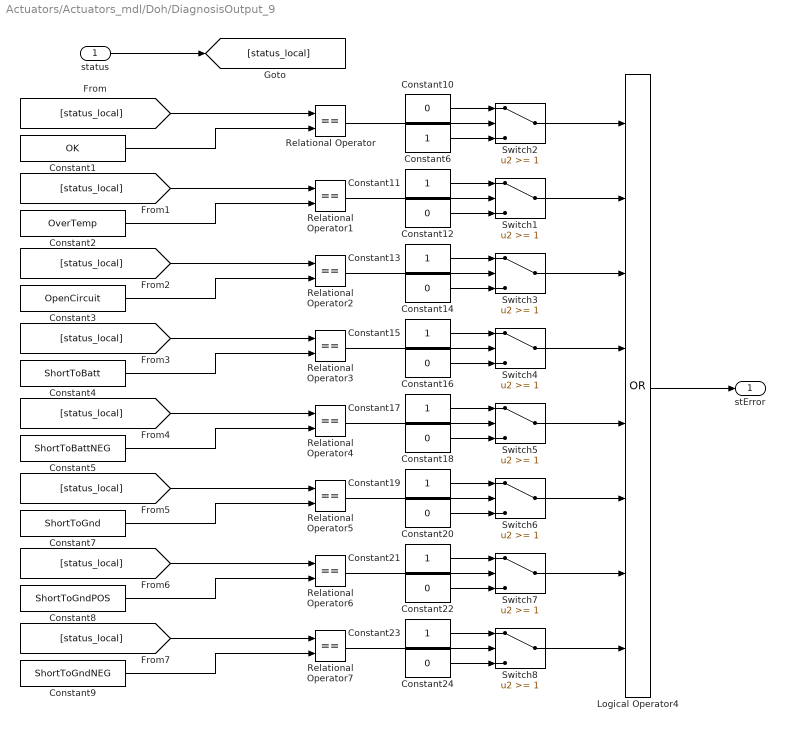
== system Actuators/Actuators_mdl/Doh/DiagnosisOutput_9 ==
  status : Inport
  Constant1 : Constant  Value=OK
  Constant{10,12,14,16,18,20,22,24} (8 alike) : Constant  Value=0  OutDataTypeStr=boolean
  Constant{6,11,13,15,17,19,21,23} (8 alike) : Constant  OutDataTypeStr=boolean
  Constant2 : Constant  Value=OverTemp
  Constant3 : Constant  Value=OpenCircuit
  Constant4 : Constant  Value=ShortToBatt
  Constant5 : Constant  Value=ShortToBattNEG
  Constant7 : Constant  Value=ShortToGnd
  Constant8 : Constant  Value=ShortToGndPOS
  Constant9 : Constant  Value=ShortToGndNEG
  Logical Operator4 : Logic  Operator=OR  Inputs=8  AllPortsSameDT=off  OutDataTypeStr=boolean
  Relational Operator{,1..7} (8 alike) : RelationalOperator  Operator===  OutDataTypeStr=boolean
  Switch{1..8} (8 alike) : Switch  Threshold=1
  stError : Outport
  wires:
  Constant1/1 -> Relational Operator/2
  status/1 -> [status_local]
  [status_local] -> Relational Operator/1
  Constant2/1 -> Relational Operator1/2
  [status_local] -> Relational Operator1/1
  Constant3/1 -> Relational Operator2/2
  [status_local] -> Relational Operator2/1
  Constant4/1 -> Relational Operator3/2
  [status_local] -> Relational Operator3/1
  Constant5/1 -> Relational Operator4/2
  [status_local] -> Relational Operator4/1
  Constant7/1 -> Relational Operator5/2
  [status_local] -> Relational Operator5/1
  Constant8/1 -> Relational Operator6/2
  [status_local] -> Relational Operator6/1
  Constant9/1 -> Relational Operator7/2
  [status_local] -> Relational Operator7/1
  Relational Operator/1 -> Switch2/2
  Constant6/1 -> Switch2/3
  Logical Operator4/1 -> stError/1
  Constant10/1 -> Switch2/1
  Constant12/1 -> Switch1/3
  Constant11/1 -> Switch1/1
  Relational Operator1/1 -> Switch1/2
  Constant14/1 -> Switch3/3
  Constant13/1 -> Switch3/1
  Relational Operator2/1 -> Switch3/2
  Constant16/1 -> Switch4/3
  Constant15/1 -> Switch4/1
  Relational Operator3/1 -> Switch4/2
  Constant18/1 -> Switch5/3
  Constant17/1 -> Switch5/1
  Relational Operator4/1 -> Switch5/2
  Constant20/1 -> Switch6/3
  Constant19/1 -> Switch6/1
  Relational Operator5/1 -> Switch6/2
  Constant22/1 -> Switch7/3
  Constant21/1 -> Switch7/1
  Relational Operator6/1 -> Switch7/2
  Constant24/1 -> Switch8/3
  Constant23/1 -> Switch8/1
  Relational Operator7/1 -> Switch8/2
  Switch2/1 -> Logical Operator4/1
  Switch1/1 -> Logical Operator4/2
  Switch3/1 -> Logical Operator4/3
  Switch4/1 -> Logical Operator4/4
  Switch5/1 -> Logical Operator4/5
  Switch6/1 -> Logical Operator4/6
  Switch7/1 -> Logical Operator4/7
  Switch8/1 -> Logical Operator4/8

== system Actuators/Actuators_mdl/Fps/G1_DigOut_Ctrl ==
  state : Inport
  DTC_DigOut_ctrl : DataTypeConversion  OutDataTypeStr=uint8  RndMeth=Nearest
  DTC_Out1 : DataTypeConversion  OutDataTypeStr=boolean
  FlexECU_DevLib_FcnAPI_Wrapper_SFcn : S-Function  FunctionName=ehooks_medc17flex_devlib_basic_io_fcncall  Parameters=NoInputPorts, NoOutputPorts, InputPortDataTypes, OutputPortDataTypes, CFunctionArgTypes, CFunctionName, ChannelName  EnableBusSupport=off  mask{NoInputPorts=1, NoOutputPorts=1, InputPortDataTypes=uint8, OutputPortDataTypes=uint8, CFunctionArgTypes=ret,val, CFunctionName=DevLib_Dio_Set, ChannelName=O_S_RL09}
      mask prompts: NoInputPorts "Number of input ports"; NoOutputPorts "Number of output ports"; InputPortDataTypes "Input port data types"; OutputPortDataTypes "Output port data types"; CFunctionArgTypes "C function argument types"; CFunctionName "C function name"; ChannelName "Channel (pin) name"
      mask Display: disp('EHOOKS FlexECU\nDevLib Wrapper\nS-Function')
  status : Outport
  wires:
  DTC_Out1/1 -> status/1
  FlexECU_DevLib_FcnAPI_Wrapper_SFcn/1 -> DTC_Out1/1
  state/1 -> DTC_DigOut_ctrl/1
  DTC_DigOut_ctrl/1 -> FlexECU_DevLib_FcnAPI_Wrapper_SFcn/1

== system Actuators/Actuators_mdl/Fps/G1_DigOut_GetError ==
  DTC_DigOut_GetError : DataTypeConversion  OutDataTypeStr=single
  FlexECU_DevLib_FcnAPI_Wrapper_SFcn : S-Function  FunctionName=ehooks_medc17flex_devlib_basic_io_fcncall  Parameters=NoInputPorts, NoOutputPorts, InputPortDataTypes, OutputPortDataTypes, CFunctionArgTypes, CFunctionName, ChannelName  EnableBusSupport=off  mask{NoInputPorts=0, NoOutputPorts=1, InputPortDataTypes=, OutputPortDataTypes=uint8, CFunctionArgTypes=ret, CFunctionName=DevLib_DioSet_GetError, ChannelName=O_S_RL09}
      mask prompts: NoInputPorts "Number of input ports"; NoOutputPorts "Number of output ports"; InputPortDataTypes "Input port data types"; OutputPortDataTypes "Output port data types"; CFunctionArgTypes "C function argument types"; CFunctionName "C function name"; ChannelName "Channel (pin) name"
      mask Display: disp('EHOOKS FlexECU\nDevLib Wrapper\nS-Function')
  status : Outport
  wires:
  FlexECU_DevLib_FcnAPI_Wrapper_SFcn/1 -> DTC_DigOut_GetError/1
  DTC_DigOut_GetError/1 -> status/1

== system Actuators/Actuators_mdl/Icc/EdgeFalling ==
  signal : Inport
  Detect Decrease : simulink/Logic and Bit Operations/Detect Decrease  vinit=0.0
  return : Outport
  wires:
  signal/1 -> Detect Decrease/1
  Detect Decrease/1 -> return/1

== system Actuators/Actuators_mdl/Icc/EdgeRising ==
  signal : Inport
  Detect Increase : simulink/Logic and Bit Operations/Detect Increase  vinit=0.0
  return : Outport
  wires:
  signal/1 -> Detect Increase/1
  Detect Increase/1 -> return/1

== system Actuators/Actuators_mdl/Icc/G1_IGN_SetParam_for_PFI ==
  szout_w : Inport
  szfuba_w : Inport  Port=2
  offz_w : Inport  Port=3
  IGN_zwcalcar_1 : Inport  Port=4
  IGN_zwcalcar_2 : Inport  Port=5
  IGN_zwcalcar_3 : Inport  Port=6
  IGN_zwcalcar_4 : Inport  Port=7
  IGN_zwcalcar_5 : Inport  Port=8
  IGN_zwcalcar_6 : Inport  Port=9
  IGN_zwcalcar_7 : Inport  Port=10
  IGN_zwcalcar_8 : Inport  Port=11
  IGN_fubaanz : Inport  Port=12
  DTC_IGN_fubaanz : DataTypeConversion  OutDataTypeStr=uint8  RndMeth=Nearest
  DTC_IGN_offz_w : DataTypeConversion  OutDataTypeStr=uint16  RndMeth=Nearest
  DTC_IGN_szfuba_w : DataTypeConversion  OutDataTypeStr=uint16  RndMeth=Nearest
  DTC_IGN_szout_w : DataTypeConversion  OutDataTypeStr=uint16  RndMeth=Nearest
  DTC_IGN_zwcalcar4 : DataTypeConversion  OutDataTypeStr=int8  RndMeth=Nearest
  DTC_IGN_zwcalcar_{1..3,5..8} (7 alike) : DataTypeConversion  OutDataTypeStr=int8  RndMeth=Nearest
  DTC_PFI_CdrvError : DataTypeConversion  OutDataTypeStr=single
  FlexECU_SFcn_PFI_Ign : S-Function  FunctionName=ehooks_medc17flex_devlib_ign_struct_fcncall  Parameters=NoInputPorts, NoOutputPorts, InputPortDataTypes, OutputPortDataTypes, CFunctionArgTypes, CFunctionName, StructMemberNames, StructTypeName, InputPortDataWidths, OutputPortDataWidths  EnableBusSupport=off  mask{NoInputPorts=5, NoOutputPorts=1, InputPortDataTypes=uint16, uint16, uint16, int8,uint8, OutputPortDataTypes=uint8, CFunctionArgTypes=ret,val, val, val, refin, val, CFunctionName=IgnCl_PfiSetParam, StructMemberNames=szout_w, szfuba_w, offz_w, zwcalcar, fubaanz, StructTypeName=IgnClInterface_type, InputPortDataWidths=1,1,1,8,1, OutputPortDataWidths=1}
      mask prompts: NoInputPorts "Number of input ports"; NoOutputPorts "Number of output ports"; InputPortDataTypes "Input port data types"; OutputPortDataTypes "Output port data types"; CFunctionArgTypes "C function argument types"; CFunctionName "C function name"; StructMemberNames "Structure member names"; StructTypeName "Structure type name"; InputPortDataWidths "Input port widths"; OutputPortDataWidths "Output port widths"
      mask Display: disp('EHOOKS FlexECU\nDevLib Wrapper\nS-Function')
  Mux : Mux  Inputs=8
  status : Outport
  wires:
  DTC_PFI_CdrvError/1 -> status/1
  FlexECU_SFcn_PFI_Ign/1 -> DTC_PFI_CdrvError/1
  DTC_IGN_offz_w/1 -> FlexECU_SFcn_PFI_Ign/3
  szout_w/1 -> DTC_IGN_szout_w/1
  DTC_IGN_zwcalcar_1/1 -> Mux/1
  Mux/1 -> FlexECU_SFcn_PFI_Ign/4  "tez_xxx"
  szfuba_w/1 -> DTC_IGN_szfuba_w/1
  DTC_IGN_szfuba_w/1 -> FlexECU_SFcn_PFI_Ign/2
  offz_w/1 -> DTC_IGN_offz_w/1
  IGN_zwcalcar_1/1 -> DTC_IGN_zwcalcar_1/1
  DTC_IGN_fubaanz/1 -> FlexECU_SFcn_PFI_Ign/5
  DTC_IGN_zwcalcar_2/1 -> Mux/2
  IGN_zwcalcar_2/1 -> DTC_IGN_zwcalcar_2/1
  DTC_IGN_zwcalcar_3/1 -> Mux/3
  IGN_zwcalcar_3/1 -> DTC_IGN_zwcalcar_3/1
  DTC_IGN_zwcalcar4/1 -> Mux/4
  IGN_zwcalcar_4/1 -> DTC_IGN_zwcalcar4/1
  DTC_IGN_zwcalcar_5/1 -> Mux/5
  IGN_zwcalcar_5/1 -> DTC_IGN_zwcalcar_5/1
  DTC_IGN_zwcalcar_6/1 -> Mux/6
  IGN_zwcalcar_6/1 -> DTC_IGN_zwcalcar_6/1
  DTC_IGN_zwcalcar_7/1 -> Mux/7
  IGN_zwcalcar_7/1 -> DTC_IGN_zwcalcar_7/1
  DTC_IGN_zwcalcar_8/1 -> Mux/8
  IGN_zwcalcar_8/1 -> DTC_IGN_zwcalcar_8/1
  IGN_fubaanz/1 -> DTC_IGN_fubaanz/1
  DTC_IGN_szout_w/1 -> FlexECU_SFcn_PFI_Ign/1

== system Actuators/Actuators_mdl/Icc/IGN_FadeOut_Immediate ==
  FlexECU_SFcn_Frm_CAN_Init : S-Function  Priority=48  FunctionName=ehooks_medc17flex_devlib_CAN_Init_fcncall  Parameters=CFunctionName  EnableBusSupport=off  mask{CFunctionName=IgnCl_fadeOutImmediate}
      mask prompts: CFunctionName "C function name"
      mask Display: disp('EHOOKS FlexECU\nDevLib Wrapper\nS-Function')

== system Actuators/Actuators_mdl/Ics/G1_DigOut_Ctrl ==
  state : Inport
  DTC_DigOut_ctrl : DataTypeConversion  OutDataTypeStr=uint8  RndMeth=Nearest
  DTC_Out1 : DataTypeConversion  OutDataTypeStr=boolean
  FlexECU_DevLib_FcnAPI_Wrapper_SFcn : S-Function  FunctionName=ehooks_medc17flex_devlib_basic_io_fcncall  Parameters=NoInputPorts, NoOutputPorts, InputPortDataTypes, OutputPortDataTypes, CFunctionArgTypes, CFunctionName, ChannelName  EnableBusSupport=off  mask{NoInputPorts=1, NoOutputPorts=1, InputPortDataTypes=uint8, OutputPortDataTypes=uint8, CFunctionArgTypes=ret,val, CFunctionName=DevLib_Dio_Set, ChannelName=O_S_RL29}
      mask prompts: NoInputPorts "Number of input ports"; NoOutputPorts "Number of output ports"; InputPortDataTypes "Input port data types"; OutputPortDataTypes "Output port data types"; CFunctionArgTypes "C function argument types"; CFunctionName "C function name"; ChannelName "Channel (pin) name"
      mask Display: disp('EHOOKS FlexECU\nDevLib Wrapper\nS-Function')
  status : Outport
  wires:
  DTC_DigOut_ctrl/1 -> FlexECU_DevLib_FcnAPI_Wrapper_SFcn/1
  state/1 -> DTC_DigOut_ctrl/1
  FlexECU_DevLib_FcnAPI_Wrapper_SFcn/1 -> DTC_Out1/1
  DTC_Out1/1 -> status/1

== system Actuators/Actuators_mdl/Ics/G1_DigOut_GetError ==
  DTC_DigOut_GetError : DataTypeConversion  OutDataTypeStr=single
  FlexECU_DevLib_FcnAPI_Wrapper_SFcn : S-Function  FunctionName=ehooks_medc17flex_devlib_basic_io_fcncall  Parameters=NoInputPorts, NoOutputPorts, InputPortDataTypes, OutputPortDataTypes, CFunctionArgTypes, CFunctionName, ChannelName  EnableBusSupport=off  mask{NoInputPorts=0, NoOutputPorts=1, InputPortDataTypes=, OutputPortDataTypes=uint8, CFunctionArgTypes=ret, CFunctionName=DevLib_DioSet_GetError, ChannelName=O_S_RL29}
      mask prompts: NoInputPorts "Number of input ports"; NoOutputPorts "Number of output ports"; InputPortDataTypes "Input port data types"; OutputPortDataTypes "Output port data types"; CFunctionArgTypes "C function argument types"; CFunctionName "C function name"; ChannelName "Channel (pin) name"
      mask Display: disp('EHOOKS FlexECU\nDevLib Wrapper\nS-Function')
  status : Outport
  wires:
  DTC_DigOut_GetError/1 -> status/1
  FlexECU_DevLib_FcnAPI_Wrapper_SFcn/1 -> DTC_DigOut_GetError/1

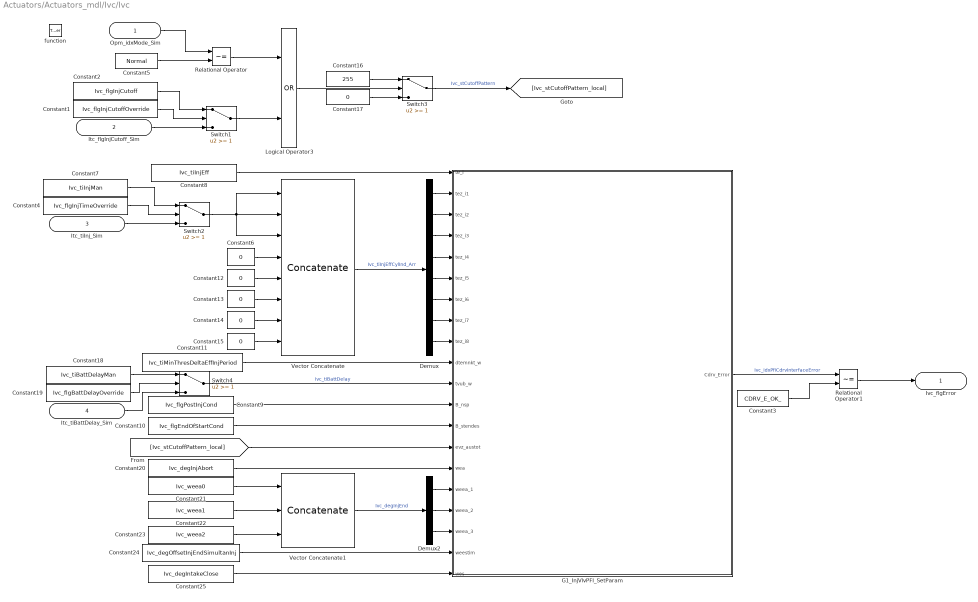
== system Actuators/Actuators_mdl/Ivc/Ivc ==
  Opm_idxMode_Sim : Inport
  Itc_flgInjCutoff_Sim : Inport  Port=2
  Itc_tiInj_Sim : Inport  Port=3
  Itc_tiBattDelay_Sim : Inport  Port=4
  function : TriggerPort  TriggerType=function-call
  Constant1 : Constant  Value=Ivc_flgInjCutoffOverride
  Constant10 : Constant  Value=Ivc_flgEndOfStartCond
  Constant11 : Constant  Value=Ivc_tiMinThresDeltaEffInjPeriod
  Constant{6,12..15} (5 alike) : Constant  Value=0  OutMin=-72  OutMax=78  OutDataTypeStr=single
  Constant16 : Constant  Value=255  OutDataTypeStr=single
  Constant17 : Constant  Value=0  OutDataTypeStr=single
  Constant18 : Constant  Value=Ivc_tiBattDelayMan
  Constant19 : Constant  Value=Ivc_flgBattDelayOverride
  Constant2 : Constant  Value=Ivc_flgInjCutoff
  Constant20 : Constant  Value=Ivc_degInjAbort
  Constant21 : Constant  Value=Ivc_weea0
  Constant22 : Constant  Value=Ivc_weea1
  Constant23 : Constant  Value=Ivc_weea2
  Constant24 : Constant  Value=Ivc_degOffsetInjEndSimultanInj
  Constant25 : Constant  Value=Ivc_degIntakeClose
  Constant3 : Constant  Value=CDRV_E_OK_
  Constant4 : Constant  Value=Ivc_flgInjTimeOverride
  Constant5 : Constant  Value=Normal
  Constant7 : Constant  Value=Ivc_tiInjMan
  Constant8 : Constant  Value=Ivc_tiInjEff
  Constant9 : Constant  Value=Ivc_flgPostInjCond
  Demux : Demux  Outputs=8
  Demux2 : Demux  Outputs=3
  G1_InjVlvPFI_SetParam : Subsystem  AncestorBlock=ehooks_medc17flex_G1_lib/Library Blocks/INJ/PFI/G1_InjVlvPFI_SetParam  mask{ChannelName=IGNORED}
      mask prompts: ChannelName "PlaceHolder_IGNORED"
      mask init:
      | ehooks_medc17flex_devlib_io_block('mask_init');
      mask TypeOptions ChannelName: IGNORED
      mask Display: image(imread('InjVlvPfi.jpg'))
  Logical Operator3 : Logic  Operator=OR  AllPortsSameDT=off  OutDataTypeStr=boolean
  Relational Operator : RelationalOperator  Operator=~=  OutDataTypeStr=boolean
  Relational Operator1 : RelationalOperator  Operator=~=  OutDataTypeStr=boolean
  Switch{1..4} (4 alike) : Switch  Threshold=1
  Vector Concatenate : Concatenate  NumInputs=8
  Vector Concatenate1 : Concatenate  NumInputs=3
  Ivc_flgError : Outport
  wires:
  Switch2/1 -> Vector Concatenate/1, Vector Concatenate/2, Vector Concatenate/3
  Constant15/1 -> Vector Concatenate/8
  Constant14/1 -> Vector Concatenate/7
  Constant13/1 -> Vector Concatenate/6
  Constant12/1 -> Vector Concatenate/5
  Constant6/1 -> Vector Concatenate/4
  Vector Concatenate/1 -> Demux/1  "Ivc_tiInjEffCylInd_Arr"
  Constant8/1 -> G1_InjVlvPFI_SetParam/1(te_i)
  Switch1/1 -> Logical Operator3/2
  Relational Operator/1 -> Logical Operator3/1
  Constant7/1 -> Switch2/1
  Constant4/1 -> Switch2/2
  Itc_tiInj_Sim/1 -> Switch2/3
  Constant3/1 -> Relational Operator1/2
  Relational Operator1/1 -> Ivc_flgError/1
  G1_InjVlvPFI_SetParam/1(Cdrv_Error) -> Relational Operator1/1  "Ivc_idxPfiCdrvInterfaceError"
  Constant5/1 -> Relational Operator/2
  Opm_idxMode_Sim/1 -> Relational Operator/1
  Itc_flgInjCutoff_Sim/1 -> Switch1/3
  Constant2/1 -> Switch1/1
  Constant1/1 -> Switch1/2
  Logical Operator3/1 -> Switch3/2
  Constant16/1 -> Switch3/1
  Constant17/1 -> Switch3/3
  Switch3/1 -> [Ivc_stCutoffPattern_local]  "Ivc_stCutoffPattern"
  Constant18/1 -> Switch4/1
  Constant19/1 -> Switch4/2
  Itc_tiBattDelay_Sim/1 -> Switch4/3
  Vector Concatenate1/1 -> Demux2/1  "Ivc_degInjEnd"
  Constant21/1 -> Vector Concatenate1/1
  Constant22/1 -> Vector Concatenate1/2
  Constant23/1 -> Vector Concatenate1/3
  Switch4/1 -> G1_InjVlvPFI_SetParam/11(tvub_w)  "Ivc_tiBattDelay"
  Constant11/1 -> G1_InjVlvPFI_SetParam/10(dtemnkt_w)
  Demux/1 -> G1_InjVlvPFI_SetParam/2(tez_i1)
  Demux/2 -> G1_InjVlvPFI_SetParam/3(tez_i2)
  Demux/3 -> G1_InjVlvPFI_SetParam/4(tez_i3)
  Demux/4 -> G1_InjVlvPFI_SetParam/5(tez_i4)
  Demux/5 -> G1_InjVlvPFI_SetParam/6(tez_i5)
  Demux/6 -> G1_InjVlvPFI_SetParam/7(tez_i6)
  Demux/7 -> G1_InjVlvPFI_SetParam/8(tez_i7)
  Demux/8 -> G1_InjVlvPFI_SetParam/9(tez_i8)
  Constant9/1 -> G1_InjVlvPFI_SetParam/12(B_nsp)
  Constant10/1 -> G1_InjVlvPFI_SetParam/13(B_stendes)
  [Ivc_stCutoffPattern_local] -> G1_InjVlvPFI_SetParam/14(evz_austot)
  Constant20/1 -> G1_InjVlvPFI_SetParam/15(wea)
  Demux2/1 -> G1_InjVlvPFI_SetParam/16(weea_1)
  Demux2/2 -> G1_InjVlvPFI_SetParam/17(weea_2)
  Demux2/3 -> G1_InjVlvPFI_SetParam/18(weea_3)
  Constant24/1 -> G1_InjVlvPFI_SetParam/19(weestim)
  Constant25/1 -> G1_InjVlvPFI_SetParam/20(wes)

== system Actuators/Actuators_mdl/Ivc/Ivc_Diag ==
  function : TriggerPort  TriggerType=function-call
  Constant3 : Constant  Value=CDRV_E_OK_
  Constant8 : Constant  Value=Ivc_flgDiagEntryCondFulfilled
  Constant9 : Constant  Value=Ivc_flgOverrunCutoff
  G1_Inj_Set_DEVE_forPFI : Subsystem  AncestorBlock=ehooks_medc17flex_G1_lib/Library Blocks/INJ/PFI/G1_Inj_Set_DEVE_forPFI  mask{ChannelName=IGNORED}
      mask prompts: ChannelName "PlaceHolder_IGNORED"
      mask help: InjVlvDeve
      mask init:
      | ehooks_medc17flex_devlib_io_block('mask_init');
      mask TypeOptions ChannelName: IGNORED
      mask Display: image(imread('InjVlvPfi.jpg'))
  Relational Operator1 : RelationalOperator  Operator=~=  OutDataTypeStr=boolean
  Ivc_flgError : Outport
  wires:
  G1_Inj_Set_DEVE_forPFI/1(Cdrv_Error) -> Relational Operator1/1  "Ivc_idxDeveCdrvInterfaceError"
  Relational Operator1/1 -> Ivc_flgError/1
  Constant3/1 -> Relational Operator1/2
  Constant9/1 -> G1_Inj_Set_DEVE_forPFI/2(B_sa)
  Constant8/1 -> G1_Inj_Set_DEVE_forPFI/1(B_desee)

== system Actuators/Actuators_mdl/Ivc/Ivc_Error ==
  Ivc : Inport
  Ivc_Diag : Inport  Port=2
  function : TriggerPort  TriggerType=function-call
  Logical Operator3 : Logic  Operator=OR  AllPortsSameDT=off  OutDataTypeStr=boolean
  Ivc_flgError : Outport
  wires:
  Logical Operator3/1 -> Ivc_flgError/1  "Ivc_flgError"
  Ivc/1 -> Logical Operator3/1
  Ivc_Diag/1 -> Logical Operator3/2

== system Actuators/Actuators_mdl/Mrs/G1_DigOut_Ctrl ==
  state : Inport
  DTC_DigOut_ctrl : DataTypeConversion  OutDataTypeStr=uint8  RndMeth=Nearest
  DTC_Out1 : DataTypeConversion  OutDataTypeStr=boolean
  FlexECU_DevLib_FcnAPI_Wrapper_SFcn : S-Function  FunctionName=ehooks_medc17flex_devlib_basic_io_fcncall  Parameters=NoInputPorts, NoOutputPorts, InputPortDataTypes, OutputPortDataTypes, CFunctionArgTypes, CFunctionName, ChannelName  EnableBusSupport=off  mask{NoInputPorts=1, NoOutputPorts=1, InputPortDataTypes=uint8, OutputPortDataTypes=uint8, CFunctionArgTypes=ret,val, CFunctionName=DevLib_Dio_Set, ChannelName=O_S_MRLY}
      mask prompts: NoInputPorts "Number of input ports"; NoOutputPorts "Number of output ports"; InputPortDataTypes "Input port data types"; OutputPortDataTypes "Output port data types"; CFunctionArgTypes "C function argument types"; CFunctionName "C function name"; ChannelName "Channel (pin) name"
      mask Display: disp('EHOOKS FlexECU\nDevLib Wrapper\nS-Function')
  status : Outport
  wires:
  DTC_DigOut_ctrl/1 -> FlexECU_DevLib_FcnAPI_Wrapper_SFcn/1
  state/1 -> DTC_DigOut_ctrl/1
  FlexECU_DevLib_FcnAPI_Wrapper_SFcn/1 -> DTC_Out1/1
  DTC_Out1/1 -> status/1
